simulink model "RVDT"  (R2021b)
settings: Solver=FixedStepDiscrete  StartTime=0.0  StopTime=10.0  FixedStep=1e-3  RelTol=1e-3
settings Model: Creator=ACH  LastModifiedBy=ACH

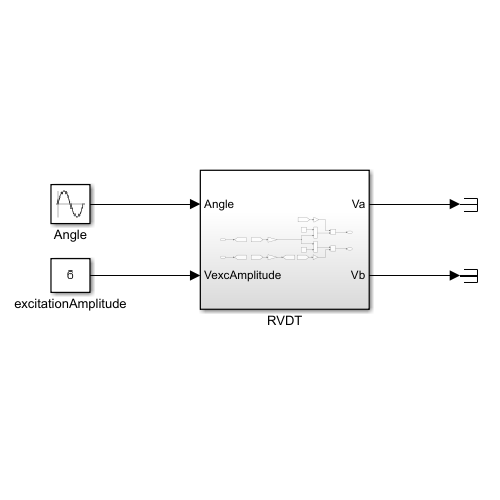
[thumbnail: Simulink's stored preview of the top-level diagram]
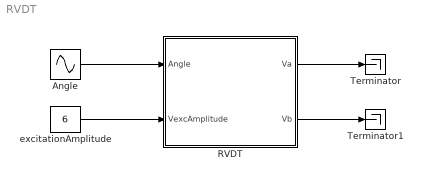
== system RVDT ==
  Angle : Sin  Amplitude=40  Frequency=2*pi*0.1  SampleTime=0
  RVDT : Subsystem
  Terminator : Terminator
  Terminator1 : Terminator
  excitationAmplitude : Constant  Value=6
  wires:
  Angle/1 -> RVDT/1(Angle)
  excitationAmplitude/1 -> RVDT/2(VexcAmplitude)
  RVDT/1(Va) -> Terminator/1
  RVDT/2(Vb) -> Terminator1/1

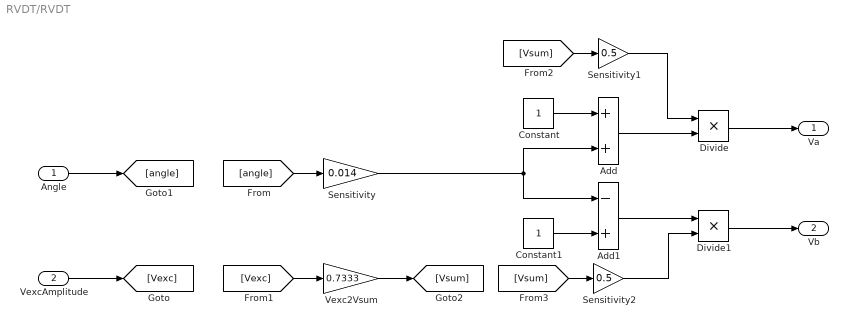
== system RVDT/RVDT ==
  Angle : Inport
  VexcAmplitude : Inport  Port=2
  Add : Sum
  Add1 : Sum  Inputs=-+
  Constant : Constant
  Constant1 : Constant
  Divide : Product  Inputs=**
  Divide1 : Product  Inputs=**
  Sensitivity : Gain  Gain=0.014
  Sensitivity1 : Gain  Gain=0.5
  Sensitivity2 : Gain  Gain=0.5
  Vexc2Vsum : Gain  Gain=0.7333
  Va : Outport
  Vb : Outport  Port=2
  wires:
  [angle] -> Sensitivity/1
  Sensitivity1/1 -> Divide/1
  Sensitivity2/1 -> Divide1/2
  Constant/1 -> Add/1
  Divide1/1 -> Vb/1
  Add/1 -> Divide/2
  Angle/1 -> [angle]
  [Vsum] -> Sensitivity1/1
  Constant1/1 -> Add1/2
  Vexc2Vsum/1 -> [Vsum]
  Sensitivity/1 -> Add1/1, Add/2
  Divide/1 -> Va/1
  [Vsum] -> Sensitivity2/1
  Add1/1 -> Divide1/1
  [Vexc] -> Vexc2Vsum/1
  VexcAmplitude/1 -> [Vexc]
